simulink model "RP_Sumo_Gamepads"  (R2019b)
settings: Solver=ode23t  StartTime=0.0  StopTime=inf  FixedStep=0.05  RelTol=1e-3  EnableMultiTasking=on
InitFcn:
  | RPInit
libraries: RoboticsPlayground x4, vexcommonlib x3, RP_Simulator_Components x3, vrlib x1
settings Model: EnablePacing=on  ExtModeTrigDuration=25  Creator=scastro  LastModifiedBy=adityaaaap
settings SolverCC: AlgebraicLoopSolver=LineSearch
settings DataIOCC: LimitDataPoints=on  ReturnWorkspaceOutputs=off
settings OptimizationCC: PassReuseOutputArgsAs=Individual arguments  MaxStackSize=64  EfficientTunableParamExpr=on
settings DebuggingCC: ParameterTunabilityLossMsg=error  UnconnectedLineMsg=none  AllowSymbolicDim=off  SFUnexpectedBacktrackingDiag=warning  SFNoUnconditionalDefaultTransitionDiag=warning  SFExecutionAtInitializationDiag=none  ArithmeticOperatorsInVariantConditions=warning
settings HardwareCC: ProdBitPerPointer=32  ProdBitPerSizeT=32  ProdBitPerPtrDiffT=32  ProdLargestAtomicInteger=Long  ProdLargestAtomicFloat=Double  ProdWordSize=32  ProdHWDeviceType=ARM Compatible->ARM Cortex
settings SFSimCC: SimUseLocalCustomCode=off  MATLABDynamicMemAlloc=off  CustomCodeUndefinedFunction=UseInterfaceOnly
settings RTWCC: SystemTargetFile=ert.tlc  HardwareBoard=ARM Cortex-based VEX Microcontroller  TLCOptions="-aInlineSetEventsForThisBaseRateFcn=TLC_FALSE -aSuppressMultiTaskScheduler=TLC_FALSE  -aRateBasedStepFcn=0"  TemplateMakefile=ert_default_tmf  GenerateReport=on  RTWUseLocalCustomCode=off  Toolchain=GNU Tools for VEX ARM Cortex  IncludeHyperlinkInReport=on  LaunchReport=on  GenerateTraceInfo=on  GenerateTraceReport=on  GenerateTraceReportSl=on  GenerateTraceReportSf=on  GenerateTraceReportEml=on
settings CodeAppCC: ForceParamTrailComments=on  IgnoreCustomStorageClasses=off  OperatorAnnotations=on  SimulinkDataObjDesc=on  SFDataObjDesc=on  InsertBlockDesc=on
settings ConfigComp: CovMetricSettings=dw  CovHtmlReporting=on  CovSaveCumulativeToWorkspaceVar=on  CovSaveSingleToWorkspaceVar=on  CovExternalEMLEnable=off  CovSFcnEnable=off
settings SimscapeCC: SimscapeNominalValues="[{\"value\":\"10\",\"unit\":\"V\"},{\"value\":\"1\",\"unit\":\"A\"},{\"value\":\"10\",\"unit\":\"N*m\"},{\"value\":\"10\",\"unit\":\"bar\"},{\"value\":\"100\",\"unit\":\"kJ/kg\"},{\"value\":\"1\",\"unit\":\"kW\"},{\"value\":\"300\",\"unit\":\"K\"},{\"value\":\"100\",\"unit\":\"cm^3/s\"},{\"value\":\"1\",\"unit\":\"kN\"},{\"value\":\"1\",\"unit\":\"g/cm^3\"},{\"value\":\"1\",\"unit\":\"l\"},{\"value\":\"1\",\"unit\":\"cm^2\"},{\"value\":\"60\",\"unit\":\"Hz\"}]"  SimscapeLogOpenViewer=on  SimscapeLogLimitData=off  SimscapeLogDataHistory=10000
settings ConfigurationSet: Description=SimMechanics 2G
settings DiagnosticsConfigSet: SimMechanicsRigidlyBoundBlock=none
settings ExplorerConfigSet: InternalSimMechanicsExplorerSettings="<ExplorerConfiguration><canonicalview>default</canonicalview><AnimationSetting><BasePlaybackSpeed>1.0</BasePlaybackSpeed><PlaybackSpeedFactor>1.0</PlaybackSpeedFactor></AnimationSetting><TilePanel><TileInfo><Tiles Columns=\"1\" Count=\"1\" Rows=\"1\"><Column Weight=\"1\"/><Row Weight=\"1\"/><Tile Height=\"1\" Width=\"1\" X=\"0\" Y=\"0\"/></Tiles></TileInfo><SceneInfo><SceneViewer><BGColor><R>0.60000002384185791</R><G>0.60000002384185791</G><B>0.60000002384185791</B></BGColor><Camera><DoPerspective>off</DoPerspective><Position><X>3.46540117628362099</X><Y>-4.48851086982872793</Y><Z>4.67527935374708381</Z></Position><Center><X>-0.00318824384245883219</X><Y>0.0743826421051177328</Y><Z>-0.042399806737498838</Z></Center><Up><X>-0.411121559241908907</X><Y>0.485309543248861219</Y><Z>0.771656471986132075</Z></Up><ViewLimDist>1</ViewLimDist><YLim>2.29173345008683382</YLim><XLim>4.12888596934658469</XLim></Camera></SceneViewer></SceneInfo></TilePanel><MechEditorPanel><Cameras/><GfxPanelCameraMap/><VideoCreator><PlaybackSpeedRatio>1.0</PlaybackSpeedRatio><FrameRate>30</FrameRate><VideoFormat>Motion JPEG AVI</VideoFormat><FrameSize>auto</FrameSize></VideoCreator></MechEditorPanel></ExplorerConfiguration>"

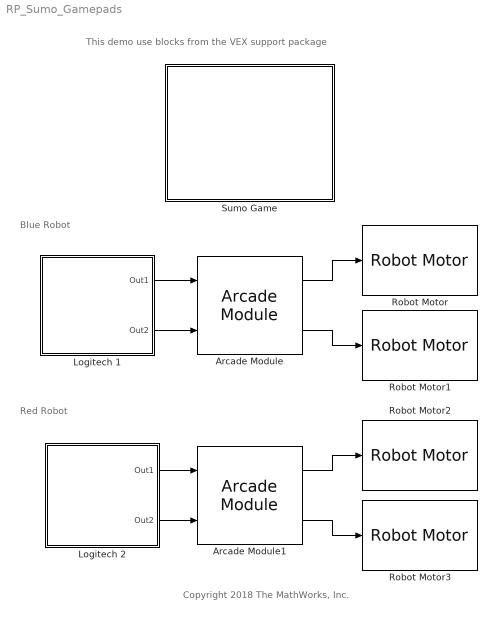
== system RP_Sumo_Gamepads ==
  note: Red Robot
  note: Blue Robot
  note: This demo use blocks from the VEX support package
  note: Copyright 2018 The MathWorks, Inc.
  Arcade Module : vexcommonlib/Arcade Module  BlockPlatform=vexarmcortex
      settings: SourceProductName=Simulink Coder Support Package for ARM Cortex-based VEX Microcontroller  SourceProductBaseCode=EC_VEX_MICRO
  Arcade Module1 : vexcommonlib/Arcade Module  BlockPlatform=vexarmcortex
      settings: SourceProductName=Simulink Coder Support Package for ARM Cortex-based VEX Microcontroller  SourceProductBaseCode=EC_VEX_MICRO
  Logitech 1 : Subsystem
      mask Display:
      | pic = imread(fullfile(codertarget.vexcommon.internal.getRootDir(),'resources','Gamepad_Controller.png'));
      | image(pic);
  Logitech 2 : Subsystem
      mask Display:
      | pic = imread(fullfile(codertarget.vexcommon.internal.getRootDir(),'resources','Gamepad_Controller.png'));
      | image(pic);
  Robot Motor : RoboticsPlayground/Basic Sensors and Actuators/Robot Motor  robotId=1  motorChoice=2
      settings: SourceProductName=Robotics Playground
  Robot Motor1 : RoboticsPlayground/Basic Sensors and Actuators/Robot Motor  robotId=1  motorChoice=1
      settings: SourceProductName=Robotics Playground
  Robot Motor2 : RoboticsPlayground/Basic Sensors and Actuators/Robot Motor  robotId=2  motorChoice=2
      settings: SourceProductName=Robotics Playground
  Robot Motor3 : RoboticsPlayground/Basic Sensors and Actuators/Robot Motor  robotId=2  motorChoice=1
      settings: SourceProductName=Robotics Playground
  Sumo Game : Subsystem  mask(RP Sumo Game){arenaLength=5, arenaWidth=5, circleRadius=1.8, difficulty=Easy, robot1Id=1, startPose1=[-0.4 0], wheelBase1=0.5, wheelRadius1=0.1, color1=[0 0 0.5], robot2Id=2, startPose2=[0.4 0], wheelBase2=0.5, wheelRadius2=0.1, color2=[0.5 0 0]}
      mask prompts: arenaLength "Length [m]"; arenaWidth "Width [m]"; circleRadius "Sumo circle radius [m]"; robot1Id "Robot ID"; startPose1 "Initial position X Y [m]"; wheelBase1 "Distance between wheels [m]"; wheelRadius1 "Wheel radius [m]"; color1 "Color [R G B]"; robot2Id "Robot ID"; startPose2 "Initial position X Y [m]"; wheelBase2 "Distance between wheels [m]"; wheelRadius2 "Wheel radius [m]"; color2 "Color"
      mask help:
      | This is a fully imlpemented simulation environment for a robot sumo game. The goal of the game is for one of the robots to push the competitor outside of the area bounded by the circle. Provide input torques to the motors through motor blocks in order to control the robot behavior.
      |
      | Motor mappings for both the robots are as follows:
      |
      | Motor 1 -> Left wheel force
      | Motor 2 -> Right wheel force
      mask init:
      | diff=get_param(gcb,'difficulty');
      | if strcmp(diff,'Medium')
      |     maxTorque=6;
      | elseif strcmp(diff,'Hard')
      |     maxTorque=9;
      | else
      |     maxTorque=3;
      | end
      | 
      | % Check robot ID's are different
      | blk=gcb;
      | id1=get_param(blk,'robot1Id');
      | id2=get_param(blk,'robot2Id');
      | 
      | if id1 == id2
      |     error('Please make sure robot ID''s are different')
      | end
      settings: CopyFcn=|
      | set_param(gcs,'InitFcn','RPInit');
      | set_param(gcs,'Solver','ode23t');
      | set_param(gcs, 'EnablePacing', 'on')
      | set_param(gcs, 'PacingRate', 1)
      mask Help: web('sumo_game.htm')
      mask TypeOptions difficulty: Easy | Medium | Hard
      mask DialogControl Container5 Prompt: Game settings
      mask DialogControl Container8 Prompt: Robot 1 settings
      mask DialogControl Container9 Prompt: Robot 2 settings
      mask Display:
      | color('white');
      | plot([100,100,100,100]*1,[100,100,100,100]*1);
      | plot([100,100,100,100]*0,[100,100,100,100]*0);
      | image('SumoGame.PNG')
      | color('blue');
      | id=eval(get_param(gcb,'robot1Id'));
      | text(99, 92, ['Robot 1 ID: ' num2str(id)], 'horizontalAlignment', 'right');
      | id=eval(get_param(gcb,'robot2Id'));
      | text(99, 82, ['Robot 2 ID: ' num2str(id)], 'horizontalAlignment', 'right');
  wires:
  Logitech 1/1(Out1) -> Arcade Module/1
  Logitech 1/2(Out2) -> Arcade Module/2
  Logitech 2/1(Out1) -> Arcade Module1/1
  Logitech 2/2(Out2) -> Arcade Module1/2
  Arcade Module/1 -> Robot Motor/1
  Arcade Module/2 -> Robot Motor1/1
  Arcade Module1/1 -> Robot Motor2/1
  Arcade Module1/2 -> Robot Motor3/1

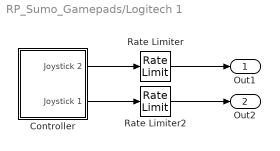
== system RP_Sumo_Gamepads/Logitech 1 ==
  Controller : Subsystem
  Rate Limiter : RateLimiter  RisingSlewLimit=1.2*127  FallingSlewLimit=-1.2*127  SampleTimeMode=inherited
  Rate Limiter2 : RateLimiter  RisingSlewLimit=1.2*127  FallingSlewLimit=-1.2*127  SampleTimeMode=inherited
  Out1 : Outport  VectorParamsAs1DForOutWhenUnconnected=off
  Out2 : Outport  Port=2  VectorParamsAs1DForOutWhenUnconnected=off
  wires:
  Rate Limiter2/1 -> Out2/1
  Rate Limiter/1 -> Out1/1
  Controller/2(Joystick 1) -> Rate Limiter2/1
  Controller/1(Joystick 2) -> Rate Limiter/1

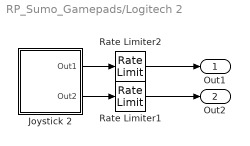
== system RP_Sumo_Gamepads/Logitech 2 ==
  Joystick 2 : Subsystem
  Rate Limiter1 : RateLimiter  RisingSlewLimit=1.2*127  FallingSlewLimit=-1.2*127  SampleTimeMode=inherited
  Rate Limiter2 : RateLimiter  RisingSlewLimit=1.2*127  FallingSlewLimit=-1.2*127  SampleTimeMode=inherited
  Out1 : Outport  VectorParamsAs1DForOutWhenUnconnected=off
  Out2 : Outport  Port=2  VectorParamsAs1DForOutWhenUnconnected=off
  wires:
  Rate Limiter1/1 -> Out2/1
  Rate Limiter2/1 -> Out1/1
  Joystick 2/1(Out1) -> Rate Limiter2/1
  Joystick 2/2(Out2) -> Rate Limiter1/1

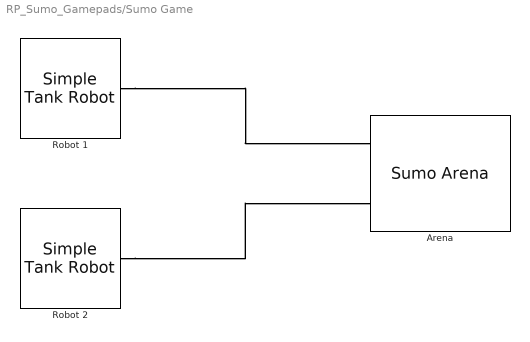
== system RP_Sumo_Gamepads/Sumo Game ==
  Arena : RP_Simulator_Components/Sumo Arena  length=arenaLength  width=arenaWidth  circleRadius=circleRadius  robotRadius1=wheelBase1/2  robotRadius2=wheelBase2/2
  Robot 1 : RP_Simulator_Components/Simple Tank Robot  robotId=1  wheelRadius=wheelRadius1  wheelBase=wheelBase1  wheelThickness=0.025  chassisThickness=0.05  startPose=startPose1  choice=off  timeConstant=0.05  wheelMass=0.1  chassisMass=1  maxWheelTorque=maxTorque  wheelColor=[0.25 0.25 0.25]  chassisColor=color1
  Robot 2 : RP_Simulator_Components/Simple Tank Robot  robotId=2  wheelRadius=wheelRadius2  wheelBase=wheelBase2  wheelThickness=0.025  chassisThickness=0.05  startPose=startPose2  choice=on  timeConstant=0.05  wheelMass=0.1  chassisMass=1  maxWheelTorque=maxTorque  wheelColor=[0.25 0.25 0.25]  chassisColor=color2
  connections:
  Robot 2/RConn1 -- Arena/LConn2
  Robot 1/RConn1 -- Arena/LConn1

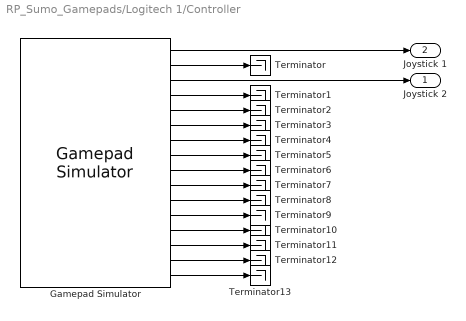
== system RP_Sumo_Gamepads/Logitech 1/Controller ==
  Gamepad Simulator : vexcommonlib/Gamepad Simulator  WhichPad=Logitech Gamepad  JoyId=1  BlockPlatform=vexarmcortex
      settings: SourceProductName=Simulink Coder Support Package for ARM Cortex-based VEX Microcontroller  SourceProductBaseCode=EC_VEX_MICRO
  Terminator{,1..13} (14 alike) : Terminator
  Joystick 2 : Outport  VectorParamsAs1DForOutWhenUnconnected=off
  Joystick 1 : Outport  Port=2  VectorParamsAs1DForOutWhenUnconnected=off
  wires:
  Gamepad Simulator/3 -> Joystick 2/1
  Gamepad Simulator/1 -> Joystick 1/1
  Gamepad Simulator/2 -> Terminator/1
  Gamepad Simulator/4 -> Terminator1/1
  Gamepad Simulator/5 -> Terminator2/1
  Gamepad Simulator/6 -> Terminator3/1
  Gamepad Simulator/7 -> Terminator4/1
  Gamepad Simulator/8 -> Terminator5/1
  Gamepad Simulator/9 -> Terminator6/1
  Gamepad Simulator/10 -> Terminator7/1
  Gamepad Simulator/11 -> Terminator8/1
  Gamepad Simulator/12 -> Terminator9/1
  Gamepad Simulator/13 -> Terminator10/1
  Gamepad Simulator/14 -> Terminator11/1
  Gamepad Simulator/15 -> Terminator12/1
  Gamepad Simulator/16 -> Terminator13/1

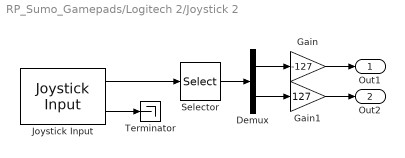
== system RP_Sumo_Gamepads/Logitech 2/Joystick 2 ==
  Demux : Demux  Outputs=2
  Gain : Gain  Gain=-127
  Gain1 : Gain  Gain=127
  Joystick Input : vrlib/Joystick Input  joyid=2  adjustports=on  forcefeed=off
      settings: SourceProductBaseCode=VR
  Selector : Selector  InputPortWidth=4  IndexOptions=Index vector (dialog)  Indices=[2 3]  OutputSizes=1
  Terminator : Terminator
  Out1 : Outport  VectorParamsAs1DForOutWhenUnconnected=off
  Out2 : Outport  Port=2  VectorParamsAs1DForOutWhenUnconnected=off
  wires:
  Gain1/1 -> Out2/1
  Gain/1 -> Out1/1
  Demux/2 -> Gain1/1
  Demux/1 -> Gain/1
  Selector/1 -> Demux/1
  Joystick Input/1 -> Selector/1
  Joystick Input/2 -> Terminator/1
